simulink model "Campus_Power_System_updated"  (R2024a)
settings: Solver=daessc  StartTime=0.0  StopTime=1  RelTol=1e-3
libraries: spsThreePhaseVIMeasurementLib x57, spsThreePhaseTransformerTwoWindingsLib x56, spsThreePhaseSeriesRLCLoadLib x55, spsThreePhasePISectionLineLib x54, spsThreePhaseBreakerLib x9, spsCurrentMeasurementLib x3, spsMultimeterLib x1, spsThreePhaseSourceLib x1, spsThreePhaseFaultLib x1, sps_lib x1
(part 3 of 3)

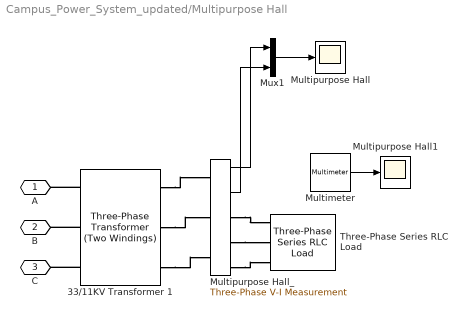
== system Campus_Power_System_updated/Multipurpose Hall ==
  33/11KV Transformer 1 : spsThreePhaseTransformerTwoWindingsLib/Three-Phase Transformer (Two Windings)  Winding1Connection=Yg  Winding2Connection=Yg  CoreType=Three single-phase transformers  SetSaturation=off  Hysteresis=off  DataFile='hysteresis'  SetInitialFlux=off  Measurements=None  UNITS=pu  NominalPower=[ 250e6 , 50 ]  Winding1=[33e3 , 0.002 , 0.08 ]  Winding2=[ 11e3 , 0.002 , 0.08 ]  Rm=500  Lm=500  L0=0.5  Saturation=[ 0,0 ; 0.0024,1.2 ; 1.0,1.52 ]  InitialFluxes=[ 0.8 , -0.8 , 0.7 ]  BreakLoop=off  DiscreteSolver=Trapezoidal iterative  DataType=off  TransfoNumber=1
  Multimeter : spsMultimeterLib/Multimeter  L=21  sel=[4 5 6]  yselected={}  Gain=[1 1 1]  OutputType=Complex  PlotAtSimulationStop=off  PhasorSimulation=off
  Multipurpose Hall : Scope
  Multipurpose Hall1 : Scope
  Multipurpose Hall_ : spsThreePhaseVIMeasurementLib/Three-Phase V-I Measurement  VoltageMeasurement=phase-to-ground  SetLabelV=off  LabelV=Vabc  Vpu=off  VpuLL=off  CurrentMeasurement=yes  SetLabelI=off  LabelI=Iabc  Ipu=off  Pbase=100e6  Vbase=500e3  OutputType=Complex  PhasorSimulation=off  PSBequivalent=0
  Mux1 : Mux  Inputs=2
  Three-Phase Series RLC Load : spsThreePhaseSeriesRLCLoadLib/Three-Phase Series RLC Load  LConnTagsString=A|B|C  Configuration=Y (grounded)  NominalVoltage=230  Vabc=[1e3 1e3 1e3]  Vabcp=[1e3 1e3 1e3]  NominalFrequency=50  UnbalancedPower=off  ActivePower=120e3  InductivePower=100  CapacitivePower=100  Pabc=[10e3 9e3 11e3]  QLabc=[100 90 110]  QCabc=[100 90 110]  Pabcp=[10e3 9e3 11e3]  QLabcp=[100 90 110]  QCabcp=[100 90 110]  Measurements=Branch currents  LoadType=constant Z
  A : PMIOPort  Side=Left
  B : PMIOPort  Port=2  Side=Left
  C : PMIOPort  Port=3  Side=Left
  wires:
  Multipurpose Hall_/2 -> Mux1/2
  Multipurpose Hall_/1 -> Mux1/1
  Mux1/1 -> Multipurpose Hall/1
  Multimeter/1 -> Multipurpose Hall1/1
  connections:
  33/11KV Transformer 1/RConn3 -- Multipurpose Hall_/LConn3
  33/11KV Transformer 1/RConn1 -- Multipurpose Hall_/LConn1
  Multipurpose Hall_/RConn2 -- Three-Phase Series RLC Load/LConn2
  Multipurpose Hall_/RConn3 -- Three-Phase Series RLC Load/LConn3
  33/11KV Transformer 1/RConn2 -- Multipurpose Hall_/LConn2
  Multipurpose Hall_/RConn1 -- Three-Phase Series RLC Load/LConn1
  33/11KV Transformer 1/LConn1 -- A/RConn1
  33/11KV Transformer 1/LConn3 -- C/RConn1
  33/11KV Transformer 1/LConn2 -- B/RConn1

== system Campus_Power_System_updated/Ogenge Odo ==
  33/11KV Transformer 1 : spsThreePhaseTransformerTwoWindingsLib/Three-Phase Transformer (Two Windings)  Winding1Connection=Yg  Winding2Connection=Yg  CoreType=Three single-phase transformers  SetSaturation=off  Hysteresis=off  DataFile='hysteresis'  SetInitialFlux=off  Measurements=None  UNITS=pu  NominalPower=[ 250e6 , 50 ]  Winding1=[33e3 , 0.002 , 0.08 ]  Winding2=[ 11e3 , 0.002 , 0.08 ]  Rm=500  Lm=500  L0=0.5  Saturation=[ 0,0 ; 0.0024,1.2 ; 1.0,1.52 ]  InitialFluxes=[ 0.8 , -0.8 , 0.7 ]  BreakLoop=off  DiscreteSolver=Trapezoidal iterative  DataType=off  TransfoNumber=1
  BUS1 : spsThreePhaseVIMeasurementLib/Three-Phase V-I Measurement  VoltageMeasurement=phase-to-ground  SetLabelV=off  LabelV=Vabc  Vpu=off  VpuLL=off  CurrentMeasurement=yes  SetLabelI=off  LabelI=Iabc  Ipu=off  Pbase=100e6  Vbase=500e3  OutputType=Complex  PhasorSimulation=off  PSBequivalent=0
  Mux1 : Mux  Inputs=2
  Scope1 : Scope
  Three-Phase Series RLC Load : spsThreePhaseSeriesRLCLoadLib/Three-Phase Series RLC Load  LConnTagsString=A|B|C  Configuration=Y (grounded)  NominalVoltage=1000  Vabc=[1e3 1e3 1e3]  Vabcp=[1e3 1e3 1e3]  NominalFrequency=60  UnbalancedPower=off  ActivePower=10e3  InductivePower=100  CapacitivePower=100  Pabc=[10e3 9e3 11e3]  QLabc=[100 90 110]  QCabc=[100 90 110]  Pabcp=[10e3 9e3 11e3]  QLabcp=[100 90 110]  QCabcp=[100 90 110]  Measurements=None  LoadType=constant Z
  A : PMIOPort  Side=Left
  B : PMIOPort  Port=2  Side=Left
  C : PMIOPort  Port=3  Side=Left
  wires:
  BUS1/2 -> Mux1/2
  BUS1/1 -> Mux1/1
  Mux1/1 -> Scope1/1
  connections:
  33/11KV Transformer 1/RConn3 -- BUS1/LConn3
  33/11KV Transformer 1/RConn1 -- BUS1/LConn1
  BUS1/RConn2 -- Three-Phase Series RLC Load/LConn2
  BUS1/RConn3 -- Three-Phase Series RLC Load/LConn3
  33/11KV Transformer 1/RConn2 -- BUS1/LConn2
  BUS1/RConn1 -- Three-Phase Series RLC Load/LConn1
  33/11KV Transformer 1/LConn1 -- A/RConn1
  33/11KV Transformer 1/LConn3 -- C/RConn1
  33/11KV Transformer 1/LConn2 -- B/RConn1

== system Campus_Power_System_updated/Ozukar Road ==
  33/11KV Transformer 1 : spsThreePhaseTransformerTwoWindingsLib/Three-Phase Transformer (Two Windings)  Winding1Connection=Yg  Winding2Connection=Yg  CoreType=Three single-phase transformers  SetSaturation=off  Hysteresis=off  DataFile='hysteresis'  SetInitialFlux=off  Measurements=None  UNITS=pu  NominalPower=[ 250e6 , 50 ]  Winding1=[33e3 , 0.002 , 0.08 ]  Winding2=[ 11e3 , 0.002 , 0.08 ]  Rm=500  Lm=500  L0=0.5  Saturation=[ 0,0 ; 0.0024,1.2 ; 1.0,1.52 ]  InitialFluxes=[ 0.8 , -0.8 , 0.7 ]  BreakLoop=off  DiscreteSolver=Trapezoidal iterative  DataType=off  TransfoNumber=1
  BUS1 : spsThreePhaseVIMeasurementLib/Three-Phase V-I Measurement  VoltageMeasurement=phase-to-ground  SetLabelV=off  LabelV=Vabc  Vpu=off  VpuLL=off  CurrentMeasurement=yes  SetLabelI=off  LabelI=Iabc  Ipu=off  Pbase=100e6  Vbase=500e3  OutputType=Complex  PhasorSimulation=off  PSBequivalent=0
  Mux1 : Mux  Inputs=2
  Scope1 : Scope
  Three-Phase Series RLC Load : spsThreePhaseSeriesRLCLoadLib/Three-Phase Series RLC Load  LConnTagsString=A|B|C  Configuration=Y (grounded)  NominalVoltage=1000  Vabc=[1e3 1e3 1e3]  Vabcp=[1e3 1e3 1e3]  NominalFrequency=60  UnbalancedPower=off  ActivePower=10e3  InductivePower=100  CapacitivePower=100  Pabc=[10e3 9e3 11e3]  QLabc=[100 90 110]  QCabc=[100 90 110]  Pabcp=[10e3 9e3 11e3]  QLabcp=[100 90 110]  QCabcp=[100 90 110]  Measurements=None  LoadType=constant Z
  A : PMIOPort  Side=Left
  B : PMIOPort  Port=2  Side=Left
  C : PMIOPort  Port=3  Side=Left
  wires:
  BUS1/2 -> Mux1/2
  BUS1/1 -> Mux1/1
  Mux1/1 -> Scope1/1
  connections:
  33/11KV Transformer 1/RConn3 -- BUS1/LConn3
  33/11KV Transformer 1/RConn1 -- BUS1/LConn1
  BUS1/RConn2 -- Three-Phase Series RLC Load/LConn2
  BUS1/RConn3 -- Three-Phase Series RLC Load/LConn3
  33/11KV Transformer 1/RConn2 -- BUS1/LConn2
  BUS1/RConn1 -- Three-Phase Series RLC Load/LConn1
  33/11KV Transformer 1/LConn1 -- A/RConn1
  33/11KV Transformer 1/LConn3 -- C/RConn1
  33/11KV Transformer 1/LConn2 -- B/RConn1

== system Campus_Power_System_updated/Place of worship ==
  33/11KV Transformer 1 : spsThreePhaseTransformerTwoWindingsLib/Three-Phase Transformer (Two Windings)  Winding1Connection=Yg  Winding2Connection=Yg  CoreType=Three single-phase transformers  SetSaturation=off  Hysteresis=off  DataFile='hysteresis'  SetInitialFlux=off  Measurements=None  UNITS=pu  NominalPower=[ 250e6 , 50 ]  Winding1=[33e3 , 0.002 , 0.08 ]  Winding2=[ 11e3 , 0.002 , 0.08 ]  Rm=500  Lm=500  L0=0.5  Saturation=[ 0,0 ; 0.0024,1.2 ; 1.0,1.52 ]  InitialFluxes=[ 0.8 , -0.8 , 0.7 ]  BreakLoop=off  DiscreteSolver=Trapezoidal iterative  DataType=off  TransfoNumber=1
  Mux1 : Mux  Inputs=2
  Place of worship : Scope
  Place of worship_ : spsThreePhaseVIMeasurementLib/Three-Phase V-I Measurement  VoltageMeasurement=phase-to-ground  SetLabelV=off  LabelV=Vabc  Vpu=off  VpuLL=off  CurrentMeasurement=yes  SetLabelI=off  LabelI=Iabc  Ipu=off  Pbase=100e6  Vbase=500e3  OutputType=Complex  PhasorSimulation=off  PSBequivalent=0
  Three-Phase Series RLC Load : spsThreePhaseSeriesRLCLoadLib/Three-Phase Series RLC Load  LConnTagsString=A|B|C  Configuration=Y (grounded)  NominalVoltage=220  Vabc=[1e3 1e3 1e3]  Vabcp=[1e3 1e3 1e3]  NominalFrequency=50  UnbalancedPower=off  ActivePower=50e3  InductivePower=100  CapacitivePower=100  Pabc=[10e3 9e3 11e3]  QLabc=[100 90 110]  QCabc=[100 90 110]  Pabcp=[10e3 9e3 11e3]  QLabcp=[100 90 110]  QCabcp=[100 90 110]  Measurements=None  LoadType=constant Z
  A : PMIOPort  Side=Left
  B : PMIOPort  Port=2  Side=Left
  C : PMIOPort  Port=3  Side=Left
  wires:
  Place of worship_/2 -> Mux1/2
  Place of worship_/1 -> Mux1/1
  Mux1/1 -> Place of worship/1
  connections:
  33/11KV Transformer 1/RConn3 -- Place of worship_/LConn3
  33/11KV Transformer 1/RConn1 -- Place of worship_/LConn1
  Place of worship_/RConn2 -- Three-Phase Series RLC Load/LConn2
  Place of worship_/RConn3 -- Three-Phase Series RLC Load/LConn3
  33/11KV Transformer 1/RConn2 -- Place of worship_/LConn2
  Place of worship_/RConn1 -- Three-Phase Series RLC Load/LConn1
  33/11KV Transformer 1/LConn1 -- A/RConn1
  33/11KV Transformer 1/LConn3 -- C/RConn1
  33/11KV Transformer 1/LConn2 -- B/RConn1

== system Campus_Power_System_updated/Professor's Quarters ==
  33/11KV Transformer 1 : spsThreePhaseTransformerTwoWindingsLib/Three-Phase Transformer (Two Windings)  Winding1Connection=Yg  Winding2Connection=Yg  CoreType=Three single-phase transformers  SetSaturation=off  Hysteresis=off  DataFile='hysteresis'  SetInitialFlux=off  Measurements=None  UNITS=pu  NominalPower=[ 250e6 , 50 ]  Winding1=[33e3 , 0.002 , 0.08 ]  Winding2=[ 11e3 , 0.002 , 0.08 ]  Rm=500  Lm=500  L0=0.5  Saturation=[ 0,0 ; 0.0024,1.2 ; 1.0,1.52 ]  InitialFluxes=[ 0.8 , -0.8 , 0.7 ]  BreakLoop=off  DiscreteSolver=Trapezoidal iterative  DataType=off  TransfoNumber=1
  BUS1 : spsThreePhaseVIMeasurementLib/Three-Phase V-I Measurement  VoltageMeasurement=phase-to-ground  SetLabelV=off  LabelV=Vabc  Vpu=off  VpuLL=off  CurrentMeasurement=yes  SetLabelI=off  LabelI=Iabc  Ipu=off  Pbase=100e6  Vbase=500e3  OutputType=Complex  PhasorSimulation=off  PSBequivalent=0
  Mux1 : Mux  Inputs=2
  Scope1 : Scope
  Three-Phase Series RLC Load : spsThreePhaseSeriesRLCLoadLib/Three-Phase Series RLC Load  LConnTagsString=A|B|C  Configuration=Y (grounded)  NominalVoltage=1000  Vabc=[1e3 1e3 1e3]  Vabcp=[1e3 1e3 1e3]  NominalFrequency=60  UnbalancedPower=off  ActivePower=10e3  InductivePower=100  CapacitivePower=100  Pabc=[10e3 9e3 11e3]  QLabc=[100 90 110]  QCabc=[100 90 110]  Pabcp=[10e3 9e3 11e3]  QLabcp=[100 90 110]  QCabcp=[100 90 110]  Measurements=None  LoadType=constant Z
  A : PMIOPort  Side=Left
  B : PMIOPort  Port=2  Side=Left
  C : PMIOPort  Port=3  Side=Left
  wires:
  BUS1/2 -> Mux1/2
  BUS1/1 -> Mux1/1
  Mux1/1 -> Scope1/1
  connections:
  33/11KV Transformer 1/RConn3 -- BUS1/LConn3
  33/11KV Transformer 1/RConn1 -- BUS1/LConn1
  BUS1/RConn2 -- Three-Phase Series RLC Load/LConn2
  BUS1/RConn3 -- Three-Phase Series RLC Load/LConn3
  33/11KV Transformer 1/RConn2 -- BUS1/LConn2
  BUS1/RConn1 -- Three-Phase Series RLC Load/LConn1
  33/11KV Transformer 1/LConn1 -- A/RConn1
  33/11KV Transformer 1/LConn3 -- C/RConn1
  33/11KV Transformer 1/LConn2 -- B/RConn1

== system Campus_Power_System_updated/Proposed RMU for Environmental ==
  33/11KV Transformer 1 : spsThreePhaseTransformerTwoWindingsLib/Three-Phase Transformer (Two Windings)  Winding1Connection=Yg  Winding2Connection=Yg  CoreType=Three single-phase transformers  SetSaturation=off  Hysteresis=off  DataFile='hysteresis'  SetInitialFlux=off  Measurements=None  UNITS=pu  NominalPower=[ 250e6 , 50 ]  Winding1=[33e3 , 0.002 , 0.08 ]  Winding2=[ 11e3 , 0.002 , 0.08 ]  Rm=500  Lm=500  L0=0.5  Saturation=[ 0,0 ; 0.0024,1.2 ; 1.0,1.52 ]  InitialFluxes=[ 0.8 , -0.8 , 0.7 ]  BreakLoop=off  DiscreteSolver=Trapezoidal iterative  DataType=off  TransfoNumber=1
  Mux1 : Mux  Inputs=2
  Proposed RMU for Environmental : Scope
  Proposed RMU for Environmental_ : spsThreePhaseVIMeasurementLib/Three-Phase V-I Measurement  VoltageMeasurement=phase-to-ground  SetLabelV=off  LabelV=Vabc  Vpu=off  VpuLL=off  CurrentMeasurement=yes  SetLabelI=off  LabelI=Iabc  Ipu=off  Pbase=100e6  Vbase=500e3  OutputType=Complex  PhasorSimulation=off  PSBequivalent=0
  Three-Phase Series RLC Load : spsThreePhaseSeriesRLCLoadLib/Three-Phase Series RLC Load  LConnTagsString=A|B|C  Configuration=Y (grounded)  NominalVoltage=220  Vabc=[1e3 1e3 1e3]  Vabcp=[1e3 1e3 1e3]  NominalFrequency=50  UnbalancedPower=off  ActivePower=60e3  InductivePower=100  CapacitivePower=100  Pabc=[10e3 9e3 11e3]  QLabc=[100 90 110]  QCabc=[100 90 110]  Pabcp=[10e3 9e3 11e3]  QLabcp=[100 90 110]  QCabcp=[100 90 110]  Measurements=None  LoadType=constant Z
  A : PMIOPort  Side=Left
  B : PMIOPort  Port=2  Side=Left
  C : PMIOPort  Port=3  Side=Left
  wires:
  Proposed RMU for Environmental_/2 -> Mux1/2
  Proposed RMU for Environmental_/1 -> Mux1/1
  Mux1/1 -> Proposed RMU for Environmental/1
  connections:
  33/11KV Transformer 1/RConn3 -- Proposed RMU for Environmental_/LConn3
  33/11KV Transformer 1/RConn1 -- Proposed RMU for Environmental_/LConn1
  Proposed RMU for Environmental_/RConn2 -- Three-Phase Series RLC Load/LConn2
  Proposed RMU for Environmental_/RConn3 -- Three-Phase Series RLC Load/LConn3
  33/11KV Transformer 1/RConn2 -- Proposed RMU for Environmental_/LConn2
  Proposed RMU for Environmental_/RConn1 -- Three-Phase Series RLC Load/LConn1
  33/11KV Transformer 1/LConn1 -- A/RConn1
  33/11KV Transformer 1/LConn3 -- C/RConn1
  33/11KV Transformer 1/LConn2 -- B/RConn1

== system Campus_Power_System_updated/RMU ==
  33/11KV Transformer 1 : spsThreePhaseTransformerTwoWindingsLib/Three-Phase Transformer (Two Windings)  Winding1Connection=Yg  Winding2Connection=Yg  CoreType=Three single-phase transformers  SetSaturation=off  Hysteresis=off  DataFile='hysteresis'  SetInitialFlux=off  Measurements=None  UNITS=pu  NominalPower=[ 250e6 , 50 ]  Winding1=[33e3 , 0.002 , 0.08 ]  Winding2=[ 11e3 , 0.002 , 0.08 ]  Rm=500  Lm=500  L0=0.5  Saturation=[ 0,0 ; 0.0024,1.2 ; 1.0,1.52 ]  InitialFluxes=[ 0.8 , -0.8 , 0.7 ]  BreakLoop=off  DiscreteSolver=Trapezoidal iterative  DataType=off  TransfoNumber=1
  BUS1 : spsThreePhaseVIMeasurementLib/Three-Phase V-I Measurement  VoltageMeasurement=phase-to-ground  SetLabelV=off  LabelV=Vabc  Vpu=off  VpuLL=off  CurrentMeasurement=yes  SetLabelI=off  LabelI=Iabc  Ipu=off  Pbase=100e6  Vbase=500e3  OutputType=Complex  PhasorSimulation=off  PSBequivalent=0
  Mux1 : Mux  Inputs=2
  Scope1 : Scope
  Three-Phase Series RLC Load : spsThreePhaseSeriesRLCLoadLib/Three-Phase Series RLC Load  LConnTagsString=A|B|C  Configuration=Y (grounded)  NominalVoltage=1000  Vabc=[1e3 1e3 1e3]  Vabcp=[1e3 1e3 1e3]  NominalFrequency=60  UnbalancedPower=off  ActivePower=10e3  InductivePower=100  CapacitivePower=100  Pabc=[10e3 9e3 11e3]  QLabc=[100 90 110]  QCabc=[100 90 110]  Pabcp=[10e3 9e3 11e3]  QLabcp=[100 90 110]  QCabcp=[100 90 110]  Measurements=None  LoadType=constant Z
  A : PMIOPort  Side=Left
  B : PMIOPort  Port=2  Side=Left
  C : PMIOPort  Port=3  Side=Left
  wires:
  BUS1/2 -> Mux1/2
  BUS1/1 -> Mux1/1
  Mux1/1 -> Scope1/1
  connections:
  33/11KV Transformer 1/RConn3 -- BUS1/LConn3
  33/11KV Transformer 1/RConn1 -- BUS1/LConn1
  BUS1/RConn2 -- Three-Phase Series RLC Load/LConn2
  BUS1/RConn3 -- Three-Phase Series RLC Load/LConn3
  33/11KV Transformer 1/RConn2 -- BUS1/LConn2
  BUS1/RConn1 -- Three-Phase Series RLC Load/LConn1
  33/11KV Transformer 1/LConn1 -- A/RConn1
  33/11KV Transformer 1/LConn3 -- C/RConn1
  33/11KV Transformer 1/LConn2 -- B/RConn1

== system Campus_Power_System_updated/Ransome Kuti Quarters ==
  33/11KV Transformer 1 : spsThreePhaseTransformerTwoWindingsLib/Three-Phase Transformer (Two Windings)  Winding1Connection=Yg  Winding2Connection=Yg  CoreType=Three single-phase transformers  SetSaturation=off  Hysteresis=off  DataFile='hysteresis'  SetInitialFlux=off  Measurements=None  UNITS=pu  NominalPower=[ 250e6 , 50 ]  Winding1=[33e3 , 0.002 , 0.08 ]  Winding2=[ 11e3 , 0.002 , 0.08 ]  Rm=500  Lm=500  L0=0.5  Saturation=[ 0,0 ; 0.0024,1.2 ; 1.0,1.52 ]  InitialFluxes=[ 0.8 , -0.8 , 0.7 ]  BreakLoop=off  DiscreteSolver=Trapezoidal iterative  DataType=off  TransfoNumber=1
  BUS1 : spsThreePhaseVIMeasurementLib/Three-Phase V-I Measurement  VoltageMeasurement=phase-to-ground  SetLabelV=off  LabelV=Vabc  Vpu=off  VpuLL=off  CurrentMeasurement=yes  SetLabelI=off  LabelI=Iabc  Ipu=off  Pbase=100e6  Vbase=500e3  OutputType=Complex  PhasorSimulation=off  PSBequivalent=0
  Mux1 : Mux  Inputs=2
  Scope1 : Scope
  Three-Phase Series RLC Load : spsThreePhaseSeriesRLCLoadLib/Three-Phase Series RLC Load  LConnTagsString=A|B|C  Configuration=Y (grounded)  NominalVoltage=1000  Vabc=[1e3 1e3 1e3]  Vabcp=[1e3 1e3 1e3]  NominalFrequency=60  UnbalancedPower=off  ActivePower=10e3  InductivePower=100  CapacitivePower=100  Pabc=[10e3 9e3 11e3]  QLabc=[100 90 110]  QCabc=[100 90 110]  Pabcp=[10e3 9e3 11e3]  QLabcp=[100 90 110]  QCabcp=[100 90 110]  Measurements=None  LoadType=constant Z
  A : PMIOPort  Side=Left
  B : PMIOPort  Port=2  Side=Left
  C : PMIOPort  Port=3  Side=Left
  wires:
  BUS1/2 -> Mux1/2
  BUS1/1 -> Mux1/1
  Mux1/1 -> Scope1/1
  connections:
  33/11KV Transformer 1/RConn3 -- BUS1/LConn3
  33/11KV Transformer 1/RConn1 -- BUS1/LConn1
  BUS1/RConn2 -- Three-Phase Series RLC Load/LConn2
  BUS1/RConn3 -- Three-Phase Series RLC Load/LConn3
  33/11KV Transformer 1/RConn2 -- BUS1/LConn2
  BUS1/RConn1 -- Three-Phase Series RLC Load/LConn1
  33/11KV Transformer 1/LConn1 -- A/RConn1
  33/11KV Transformer 1/LConn3 -- C/RConn1
  33/11KV Transformer 1/LConn2 -- B/RConn1

== system Campus_Power_System_updated/Science Complex N ==
  33/11KV Transformer 1 : spsThreePhaseTransformerTwoWindingsLib/Three-Phase Transformer (Two Windings)  Winding1Connection=Yg  Winding2Connection=Yg  CoreType=Three single-phase transformers  SetSaturation=off  Hysteresis=off  DataFile='hysteresis'  SetInitialFlux=off  Measurements=None  UNITS=pu  NominalPower=[ 250e6 , 50 ]  Winding1=[33e3 , 0.002 , 0.08 ]  Winding2=[ 11e3 , 0.002 , 0.08 ]  Rm=500  Lm=500  L0=0.5  Saturation=[ 0,0 ; 0.0024,1.2 ; 1.0,1.52 ]  InitialFluxes=[ 0.8 , -0.8 , 0.7 ]  BreakLoop=off  DiscreteSolver=Trapezoidal iterative  DataType=off  TransfoNumber=1
  BUS1 : spsThreePhaseVIMeasurementLib/Three-Phase V-I Measurement  VoltageMeasurement=phase-to-ground  SetLabelV=off  LabelV=Vabc  Vpu=off  VpuLL=off  CurrentMeasurement=yes  SetLabelI=off  LabelI=Iabc  Ipu=off  Pbase=100e6  Vbase=500e3  OutputType=Complex  PhasorSimulation=off  PSBequivalent=0
  Mux1 : Mux  Inputs=2
  Scope1 : Scope
  Three-Phase Series RLC Load : spsThreePhaseSeriesRLCLoadLib/Three-Phase Series RLC Load  LConnTagsString=A|B|C  Configuration=Y (grounded)  NominalVoltage=1000  Vabc=[1e3 1e3 1e3]  Vabcp=[1e3 1e3 1e3]  NominalFrequency=60  UnbalancedPower=off  ActivePower=10e3  InductivePower=100  CapacitivePower=100  Pabc=[10e3 9e3 11e3]  QLabc=[100 90 110]  QCabc=[100 90 110]  Pabcp=[10e3 9e3 11e3]  QLabcp=[100 90 110]  QCabcp=[100 90 110]  Measurements=None  LoadType=constant Z
  A : PMIOPort  Side=Left
  B : PMIOPort  Port=2  Side=Left
  C : PMIOPort  Port=3  Side=Left
  wires:
  BUS1/2 -> Mux1/2
  BUS1/1 -> Mux1/1
  Mux1/1 -> Scope1/1
  connections:
  33/11KV Transformer 1/RConn3 -- BUS1/LConn3
  33/11KV Transformer 1/RConn1 -- BUS1/LConn1
  BUS1/RConn2 -- Three-Phase Series RLC Load/LConn2
  BUS1/RConn3 -- Three-Phase Series RLC Load/LConn3
  33/11KV Transformer 1/RConn2 -- BUS1/LConn2
  BUS1/RConn1 -- Three-Phase Series RLC Load/LConn1
  33/11KV Transformer 1/LConn1 -- A/RConn1
  33/11KV Transformer 1/LConn3 -- C/RConn1
  33/11KV Transformer 1/LConn2 -- B/RConn1

== system Campus_Power_System_updated/Science Conplex S ==
  33/11KV Transformer 1 : spsThreePhaseTransformerTwoWindingsLib/Three-Phase Transformer (Two Windings)  Winding1Connection=Yg  Winding2Connection=Yg  CoreType=Three single-phase transformers  SetSaturation=off  Hysteresis=off  DataFile='hysteresis'  SetInitialFlux=off  Measurements=None  UNITS=pu  NominalPower=[ 250e6 , 50 ]  Winding1=[33e3 , 0.002 , 0.08 ]  Winding2=[ 11e3 , 0.002 , 0.08 ]  Rm=500  Lm=500  L0=0.5  Saturation=[ 0,0 ; 0.0024,1.2 ; 1.0,1.52 ]  InitialFluxes=[ 0.8 , -0.8 , 0.7 ]  BreakLoop=off  DiscreteSolver=Trapezoidal iterative  DataType=off  TransfoNumber=1
  BUS1 : spsThreePhaseVIMeasurementLib/Three-Phase V-I Measurement  VoltageMeasurement=phase-to-ground  SetLabelV=off  LabelV=Vabc  Vpu=off  VpuLL=off  CurrentMeasurement=yes  SetLabelI=off  LabelI=Iabc  Ipu=off  Pbase=100e6  Vbase=500e3  OutputType=Complex  PhasorSimulation=off  PSBequivalent=0
  Mux1 : Mux  Inputs=2
  Scope1 : Scope
  Three-Phase Series RLC Load : spsThreePhaseSeriesRLCLoadLib/Three-Phase Series RLC Load  LConnTagsString=A|B|C  Configuration=Y (grounded)  NominalVoltage=1000  Vabc=[1e3 1e3 1e3]  Vabcp=[1e3 1e3 1e3]  NominalFrequency=60  UnbalancedPower=off  ActivePower=10e3  InductivePower=100  CapacitivePower=100  Pabc=[10e3 9e3 11e3]  QLabc=[100 90 110]  QCabc=[100 90 110]  Pabcp=[10e3 9e3 11e3]  QLabcp=[100 90 110]  QCabcp=[100 90 110]  Measurements=None  LoadType=constant Z
  A : PMIOPort  Side=Left
  B : PMIOPort  Port=2  Side=Left
  C : PMIOPort  Port=3  Side=Left
  wires:
  BUS1/2 -> Mux1/2
  BUS1/1 -> Mux1/1
  Mux1/1 -> Scope1/1
  connections:
  33/11KV Transformer 1/RConn3 -- BUS1/LConn3
  33/11KV Transformer 1/RConn1 -- BUS1/LConn1
  BUS1/RConn2 -- Three-Phase Series RLC Load/LConn2
  BUS1/RConn3 -- Three-Phase Series RLC Load/LConn3
  33/11KV Transformer 1/RConn2 -- BUS1/LConn2
  BUS1/RConn1 -- Three-Phase Series RLC Load/LConn1
  33/11KV Transformer 1/LConn1 -- A/RConn1
  33/11KV Transformer 1/LConn3 -- C/RConn1
  33/11KV Transformer 1/LConn2 -- B/RConn1

== system Campus_Power_System_updated/Science complex E ==
  33/11KV Transformer 1 : spsThreePhaseTransformerTwoWindingsLib/Three-Phase Transformer (Two Windings)  Winding1Connection=Yg  Winding2Connection=Yg  CoreType=Three single-phase transformers  SetSaturation=off  Hysteresis=off  DataFile='hysteresis'  SetInitialFlux=off  Measurements=None  UNITS=pu  NominalPower=[ 250e6 , 50 ]  Winding1=[33e3 , 0.002 , 0.08 ]  Winding2=[ 11e3 , 0.002 , 0.08 ]  Rm=500  Lm=500  L0=0.5  Saturation=[ 0,0 ; 0.0024,1.2 ; 1.0,1.52 ]  InitialFluxes=[ 0.8 , -0.8 , 0.7 ]  BreakLoop=off  DiscreteSolver=Trapezoidal iterative  DataType=off  TransfoNumber=1
  BUS1 : spsThreePhaseVIMeasurementLib/Three-Phase V-I Measurement  VoltageMeasurement=phase-to-ground  SetLabelV=off  LabelV=Vabc  Vpu=off  VpuLL=off  CurrentMeasurement=yes  SetLabelI=off  LabelI=Iabc  Ipu=off  Pbase=100e6  Vbase=500e3  OutputType=Complex  PhasorSimulation=off  PSBequivalent=0
  Mux1 : Mux  Inputs=2
  Scope1 : Scope
  Three-Phase Series RLC Load : spsThreePhaseSeriesRLCLoadLib/Three-Phase Series RLC Load  LConnTagsString=A|B|C  Configuration=Y (grounded)  NominalVoltage=1000  Vabc=[1e3 1e3 1e3]  Vabcp=[1e3 1e3 1e3]  NominalFrequency=60  UnbalancedPower=off  ActivePower=10e3  InductivePower=100  CapacitivePower=100  Pabc=[10e3 9e3 11e3]  QLabc=[100 90 110]  QCabc=[100 90 110]  Pabcp=[10e3 9e3 11e3]  QLabcp=[100 90 110]  QCabcp=[100 90 110]  Measurements=None  LoadType=constant Z
  A : PMIOPort  Side=Left
  B : PMIOPort  Port=2  Side=Left
  C : PMIOPort  Port=3  Side=Left
  wires:
  BUS1/2 -> Mux1/2
  BUS1/1 -> Mux1/1
  Mux1/1 -> Scope1/1
  connections:
  33/11KV Transformer 1/RConn3 -- BUS1/LConn3
  33/11KV Transformer 1/RConn1 -- BUS1/LConn1
  BUS1/RConn2 -- Three-Phase Series RLC Load/LConn2
  BUS1/RConn3 -- Three-Phase Series RLC Load/LConn3
  33/11KV Transformer 1/RConn2 -- BUS1/LConn2
  BUS1/RConn1 -- Three-Phase Series RLC Load/LConn1
  33/11KV Transformer 1/LConn1 -- A/RConn1
  33/11KV Transformer 1/LConn3 -- C/RConn1
  33/11KV Transformer 1/LConn2 -- B/RConn1

== system Campus_Power_System_updated/Senate House (1) ==
  33/11KV Transformer 1 : spsThreePhaseTransformerTwoWindingsLib/Three-Phase Transformer (Two Windings)  Winding1Connection=Yg  Winding2Connection=Yg  CoreType=Three single-phase transformers  SetSaturation=off  Hysteresis=off  DataFile='hysteresis'  SetInitialFlux=off  Measurements=None  UNITS=pu  NominalPower=[ 250e6 , 50 ]  Winding1=[33e3 , 0.002 , 0.08 ]  Winding2=[ 11e3 , 0.002 , 0.08 ]  Rm=500  Lm=500  L0=0.5  Saturation=[ 0,0 ; 0.0024,1.2 ; 1.0,1.52 ]  InitialFluxes=[ 0.8 , -0.8 , 0.7 ]  BreakLoop=off  DiscreteSolver=Trapezoidal iterative  DataType=off  TransfoNumber=1
  BUS1 : spsThreePhaseVIMeasurementLib/Three-Phase V-I Measurement  VoltageMeasurement=phase-to-ground  SetLabelV=off  LabelV=Vabc  Vpu=off  VpuLL=off  CurrentMeasurement=yes  SetLabelI=off  LabelI=Iabc  Ipu=off  Pbase=100e6  Vbase=500e3  OutputType=Complex  PhasorSimulation=off  PSBequivalent=0
  Mux1 : Mux  Inputs=2
  Scope1 : Scope
  Three-Phase Series RLC Load : spsThreePhaseSeriesRLCLoadLib/Three-Phase Series RLC Load  LConnTagsString=A|B|C  Configuration=Y (grounded)  NominalVoltage=1000  Vabc=[1e3 1e3 1e3]  Vabcp=[1e3 1e3 1e3]  NominalFrequency=60  UnbalancedPower=off  ActivePower=10e3  InductivePower=100  CapacitivePower=100  Pabc=[10e3 9e3 11e3]  QLabc=[100 90 110]  QCabc=[100 90 110]  Pabcp=[10e3 9e3 11e3]  QLabcp=[100 90 110]  QCabcp=[100 90 110]  Measurements=None  LoadType=constant Z
  A : PMIOPort  Side=Left
  B : PMIOPort  Port=2  Side=Left
  C : PMIOPort  Port=3  Side=Left
  wires:
  BUS1/2 -> Mux1/2
  BUS1/1 -> Mux1/1
  Mux1/1 -> Scope1/1
  connections:
  33/11KV Transformer 1/RConn3 -- BUS1/LConn3
  33/11KV Transformer 1/RConn1 -- BUS1/LConn1
  BUS1/RConn2 -- Three-Phase Series RLC Load/LConn2
  BUS1/RConn3 -- Three-Phase Series RLC Load/LConn3
  33/11KV Transformer 1/RConn2 -- BUS1/LConn2
  BUS1/RConn1 -- Three-Phase Series RLC Load/LConn1
  33/11KV Transformer 1/LConn1 -- A/RConn1
  33/11KV Transformer 1/LConn3 -- C/RConn1
  33/11KV Transformer 1/LConn2 -- B/RConn1

== system Campus_Power_System_updated/Senate House (2) ==
  33/11KV Transformer 1 : spsThreePhaseTransformerTwoWindingsLib/Three-Phase Transformer (Two Windings)  Winding1Connection=Yg  Winding2Connection=Yg  CoreType=Three single-phase transformers  SetSaturation=off  Hysteresis=off  DataFile='hysteresis'  SetInitialFlux=off  Measurements=None  UNITS=pu  NominalPower=[ 250e6 , 50 ]  Winding1=[33e3 , 0.002 , 0.08 ]  Winding2=[ 11e3 , 0.002 , 0.08 ]  Rm=500  Lm=500  L0=0.5  Saturation=[ 0,0 ; 0.0024,1.2 ; 1.0,1.52 ]  InitialFluxes=[ 0.8 , -0.8 , 0.7 ]  BreakLoop=off  DiscreteSolver=Trapezoidal iterative  DataType=off  TransfoNumber=1
  BUS1 : spsThreePhaseVIMeasurementLib/Three-Phase V-I Measurement  VoltageMeasurement=phase-to-ground  SetLabelV=off  LabelV=Vabc  Vpu=off  VpuLL=off  CurrentMeasurement=yes  SetLabelI=off  LabelI=Iabc  Ipu=off  Pbase=100e6  Vbase=500e3  OutputType=Complex  PhasorSimulation=off  PSBequivalent=0
  Mux1 : Mux  Inputs=2
  Scope1 : Scope
  Three-Phase Series RLC Load : spsThreePhaseSeriesRLCLoadLib/Three-Phase Series RLC Load  LConnTagsString=A|B|C  Configuration=Y (grounded)  NominalVoltage=1000  Vabc=[1e3 1e3 1e3]  Vabcp=[1e3 1e3 1e3]  NominalFrequency=60  UnbalancedPower=off  ActivePower=10e3  InductivePower=100  CapacitivePower=100  Pabc=[10e3 9e3 11e3]  QLabc=[100 90 110]  QCabc=[100 90 110]  Pabcp=[10e3 9e3 11e3]  QLabcp=[100 90 110]  QCabcp=[100 90 110]  Measurements=None  LoadType=constant Z
  A : PMIOPort  Side=Left
  B : PMIOPort  Port=2  Side=Left
  C : PMIOPort  Port=3  Side=Left
  wires:
  BUS1/2 -> Mux1/2
  BUS1/1 -> Mux1/1
  Mux1/1 -> Scope1/1
  connections:
  33/11KV Transformer 1/RConn3 -- BUS1/LConn3
  33/11KV Transformer 1/RConn1 -- BUS1/LConn1
  BUS1/RConn2 -- Three-Phase Series RLC Load/LConn2
  BUS1/RConn3 -- Three-Phase Series RLC Load/LConn3
  33/11KV Transformer 1/RConn2 -- BUS1/LConn2
  BUS1/RConn1 -- Three-Phase Series RLC Load/LConn1
  33/11KV Transformer 1/LConn1 -- A/RConn1
  33/11KV Transformer 1/LConn3 -- C/RConn1
  33/11KV Transformer 1/LConn2 -- B/RConn1

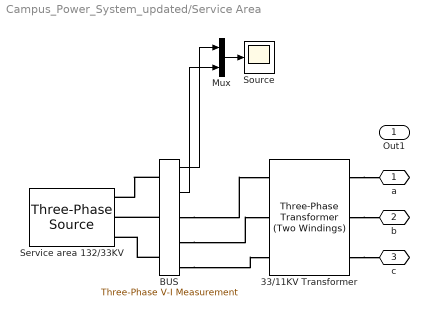
== system Campus_Power_System_updated/Service Area ==
  "33/11KV Transformer " : spsThreePhaseTransformerTwoWindingsLib/Three-Phase Transformer (Two Windings)  Winding1Connection=Yg  Winding2Connection=Yg  CoreType=Three single-phase transformers  SetSaturation=off  Hysteresis=off  DataFile='hysteresis'  SetInitialFlux=off  Measurements=None  UNITS=pu  NominalPower=[ 250e6 , 50 ]  Winding1=[33e3 , 0.002 , 0.08 ]  Winding2=[ 11e3 , 0.002 , 0.08 ]  Rm=500  Lm=500  L0=0.5  Saturation=[ 0,0 ; 0.0024,1.2 ; 1.0,1.52 ]  InitialFluxes=[ 0.8 , -0.8 , 0.7 ]  BreakLoop=off  DiscreteSolver=Trapezoidal iterative  DataType=off  TransfoNumber=1
  BUS : spsThreePhaseVIMeasurementLib/Three-Phase V-I Measurement  VoltageMeasurement=phase-to-ground  SetLabelV=off  LabelV=Vabc  Vpu=off  VpuLL=off  CurrentMeasurement=yes  SetLabelI=off  LabelI=Iabc  Ipu=off  Pbase=100e6  Vbase=500e3  OutputType=Complex  PhasorSimulation=off  PSBequivalent=0
  Mux : Mux  Inputs=2
  Service area 132/33KV : spsThreePhaseSourceLib/Three-Phase Source  InternalConnection=Yg  VoltagePhases=off  Voltage=25e3  PhaseAngle=0  Voltage_phases=[25e3 25e3 25e3]/sqrt(3)  PhaseAngles_phases=[0 -120 +120]  Frequency=50  NonIdealSource=on  SpecifyImpedance=off  Resistance=0.1  Inductance=0.01  ShortCircuitLevel=100e6  BaseVoltage=25e3  XRratio=7  BusType=swing  Pref=10e3  Qref=0  Prefabc=[10e3, 10e3, 10e3]  Qrefabc=[0, 0, 0]  Qmin=-inf  Qmax=inf
  Source : Scope
  a : PMIOPort  Side=Right
  b : PMIOPort  Port=2  Side=Right
  c : PMIOPort  Port=3  Side=Right
  Out1 : Outport
  wires:
  Mux/1 -> Source/1
  BUS/2 -> Mux/2
  BUS/1 -> Mux/1
  connections:
  BUS/RConn1 -- "33/11KV Transformer "/LConn1
  BUS/LConn2 -- Service area 132/33KV/RConn2
  "33/11KV Transformer "/RConn2 -- b/RConn1
  BUS/LConn3 -- Service area 132/33KV/RConn3
  BUS/RConn3 -- "33/11KV Transformer "/LConn3
  BUS/LConn1 -- Service area 132/33KV/RConn1
  BUS/RConn2 -- "33/11KV Transformer "/LConn2
  "33/11KV Transformer "/RConn3 -- c/RConn1
  "33/11KV Transformer "/RConn1 -- a/RConn1

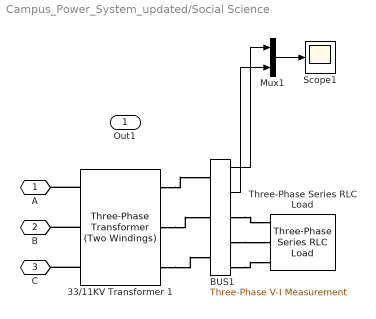
== system Campus_Power_System_updated/Social Science ==
  33/11KV Transformer 1 : spsThreePhaseTransformerTwoWindingsLib/Three-Phase Transformer (Two Windings)  Winding1Connection=Yg  Winding2Connection=Yg  CoreType=Three single-phase transformers  SetSaturation=off  Hysteresis=off  DataFile='hysteresis'  SetInitialFlux=off  Measurements=None  UNITS=pu  NominalPower=[ 250e6 , 50 ]  Winding1=[33e3 , 0.002 , 0.08 ]  Winding2=[ 11e3 , 0.002 , 0.08 ]  Rm=500  Lm=500  L0=0.5  Saturation=[ 0,0 ; 0.0024,1.2 ; 1.0,1.52 ]  InitialFluxes=[ 0.8 , -0.8 , 0.7 ]  BreakLoop=off  DiscreteSolver=Trapezoidal iterative  DataType=off  TransfoNumber=1
  BUS1 : spsThreePhaseVIMeasurementLib/Three-Phase V-I Measurement  VoltageMeasurement=phase-to-ground  SetLabelV=off  LabelV=Vabc  Vpu=off  VpuLL=off  CurrentMeasurement=yes  SetLabelI=off  LabelI=Iabc  Ipu=off  Pbase=100e6  Vbase=500e3  OutputType=Complex  PhasorSimulation=off  PSBequivalent=0
  Mux1 : Mux  Inputs=2
  Scope1 : Scope
  Three-Phase Series RLC Load : spsThreePhaseSeriesRLCLoadLib/Three-Phase Series RLC Load  LConnTagsString=A|B|C  Configuration=Y (grounded)  NominalVoltage=1000  Vabc=[1e3 1e3 1e3]  Vabcp=[1e3 1e3 1e3]  NominalFrequency=60  UnbalancedPower=off  ActivePower=10e3  InductivePower=100  CapacitivePower=100  Pabc=[10e3 9e3 11e3]  QLabc=[100 90 110]  QCabc=[100 90 110]  Pabcp=[10e3 9e3 11e3]  QLabcp=[100 90 110]  QCabcp=[100 90 110]  Measurements=None  LoadType=constant Z
  A : PMIOPort  Side=Left
  B : PMIOPort  Port=2  Side=Left
  C : PMIOPort  Port=3  Side=Left
  Out1 : Outport
  wires:
  BUS1/2 -> Mux1/2
  BUS1/1 -> Mux1/1
  Mux1/1 -> Scope1/1
  connections:
  33/11KV Transformer 1/RConn3 -- BUS1/LConn3
  33/11KV Transformer 1/RConn1 -- BUS1/LConn1
  BUS1/RConn2 -- Three-Phase Series RLC Load/LConn2
  BUS1/RConn3 -- Three-Phase Series RLC Load/LConn3
  33/11KV Transformer 1/RConn2 -- BUS1/LConn2
  BUS1/RConn1 -- Three-Phase Series RLC Load/LConn1
  33/11KV Transformer 1/LConn1 -- A/RConn1
  33/11KV Transformer 1/LConn3 -- C/RConn1
  33/11KV Transformer 1/LConn2 -- B/RConn1

== system Campus_Power_System_updated/Sport centre ==
  33/11KV Transformer 1 : spsThreePhaseTransformerTwoWindingsLib/Three-Phase Transformer (Two Windings)  Winding1Connection=Yg  Winding2Connection=Yg  CoreType=Three single-phase transformers  SetSaturation=off  Hysteresis=off  DataFile='hysteresis'  SetInitialFlux=off  Measurements=None  UNITS=pu  NominalPower=[ 250e6 , 50 ]  Winding1=[33e3 , 0.002 , 0.08 ]  Winding2=[ 11e3 , 0.002 , 0.08 ]  Rm=500  Lm=500  L0=0.5  Saturation=[ 0,0 ; 0.0024,1.2 ; 1.0,1.52 ]  InitialFluxes=[ 0.8 , -0.8 , 0.7 ]  BreakLoop=off  DiscreteSolver=Trapezoidal iterative  DataType=off  TransfoNumber=1
  BUS1 : spsThreePhaseVIMeasurementLib/Three-Phase V-I Measurement  VoltageMeasurement=phase-to-ground  SetLabelV=off  LabelV=Vabc  Vpu=off  VpuLL=off  CurrentMeasurement=yes  SetLabelI=off  LabelI=Iabc  Ipu=off  Pbase=100e6  Vbase=500e3  OutputType=Complex  PhasorSimulation=off  PSBequivalent=0
  Mux1 : Mux  Inputs=2
  Scope1 : Scope
  Three-Phase Series RLC Load : spsThreePhaseSeriesRLCLoadLib/Three-Phase Series RLC Load  LConnTagsString=A|B|C  Configuration=Y (grounded)  NominalVoltage=1000  Vabc=[1e3 1e3 1e3]  Vabcp=[1e3 1e3 1e3]  NominalFrequency=60  UnbalancedPower=off  ActivePower=10e3  InductivePower=100  CapacitivePower=100  Pabc=[10e3 9e3 11e3]  QLabc=[100 90 110]  QCabc=[100 90 110]  Pabcp=[10e3 9e3 11e3]  QLabcp=[100 90 110]  QCabcp=[100 90 110]  Measurements=None  LoadType=constant Z
  A : PMIOPort  Side=Left
  B : PMIOPort  Port=2  Side=Left
  C : PMIOPort  Port=3  Side=Left
  wires:
  BUS1/2 -> Mux1/2
  BUS1/1 -> Mux1/1
  Mux1/1 -> Scope1/1
  connections:
  33/11KV Transformer 1/RConn3 -- BUS1/LConn3
  33/11KV Transformer 1/RConn1 -- BUS1/LConn1
  BUS1/RConn2 -- Three-Phase Series RLC Load/LConn2
  BUS1/RConn3 -- Three-Phase Series RLC Load/LConn3
  33/11KV Transformer 1/RConn2 -- BUS1/LConn2
  BUS1/RConn1 -- Three-Phase Series RLC Load/LConn1
  33/11KV Transformer 1/LConn1 -- A/RConn1
  33/11KV Transformer 1/LConn3 -- C/RConn1
  33/11KV Transformer 1/LConn2 -- B/RConn1

== system Campus_Power_System_updated/Subsystem53 ==
  33/11KV Transformer 1 : spsThreePhaseTransformerTwoWindingsLib/Three-Phase Transformer (Two Windings)  Winding1Connection=Yg  Winding2Connection=Yg  CoreType=Three single-phase transformers  SetSaturation=off  Hysteresis=off  DataFile='hysteresis'  SetInitialFlux=off  Measurements=None  UNITS=pu  NominalPower=[ 250e6 , 50 ]  Winding1=[33e3 , 0.002 , 0.08 ]  Winding2=[ 11e3 , 0.002 , 0.08 ]  Rm=500  Lm=500  L0=0.5  Saturation=[ 0,0 ; 0.0024,1.2 ; 1.0,1.52 ]  InitialFluxes=[ 0.8 , -0.8 , 0.7 ]  BreakLoop=off  DiscreteSolver=Trapezoidal iterative  DataType=off  TransfoNumber=1
  BUS1 : spsThreePhaseVIMeasurementLib/Three-Phase V-I Measurement  VoltageMeasurement=phase-to-ground  SetLabelV=off  LabelV=Vabc  Vpu=off  VpuLL=off  CurrentMeasurement=yes  SetLabelI=off  LabelI=Iabc  Ipu=off  Pbase=100e6  Vbase=500e3  OutputType=Complex  PhasorSimulation=off  PSBequivalent=0
  Mux1 : Mux  Inputs=2
  Scope1 : Scope
  Three-Phase Series RLC Load : spsThreePhaseSeriesRLCLoadLib/Three-Phase Series RLC Load  LConnTagsString=A|B|C  Configuration=Y (grounded)  NominalVoltage=1000  Vabc=[1e3 1e3 1e3]  Vabcp=[1e3 1e3 1e3]  NominalFrequency=60  UnbalancedPower=off  ActivePower=10e3  InductivePower=100  CapacitivePower=100  Pabc=[10e3 9e3 11e3]  QLabc=[100 90 110]  QCabc=[100 90 110]  Pabcp=[10e3 9e3 11e3]  QLabcp=[100 90 110]  QCabcp=[100 90 110]  Measurements=None  LoadType=constant Z
  A : PMIOPort  Side=Left
  B : PMIOPort  Port=2  Side=Left
  C : PMIOPort  Port=3  Side=Left
  wires:
  BUS1/2 -> Mux1/2
  BUS1/1 -> Mux1/1
  Mux1/1 -> Scope1/1
  connections:
  33/11KV Transformer 1/RConn3 -- BUS1/LConn3
  33/11KV Transformer 1/RConn1 -- BUS1/LConn1
  BUS1/RConn2 -- Three-Phase Series RLC Load/LConn2
  BUS1/RConn3 -- Three-Phase Series RLC Load/LConn3
  33/11KV Transformer 1/RConn2 -- BUS1/LConn2
  BUS1/RConn1 -- Three-Phase Series RLC Load/LConn1
  33/11KV Transformer 1/LConn1 -- A/RConn1
  33/11KV Transformer 1/LConn3 -- C/RConn1
  33/11KV Transformer 1/LConn2 -- B/RConn1

== system Campus_Power_System_updated/Tinubu Close ==
  33/11KV Transformer 1 : spsThreePhaseTransformerTwoWindingsLib/Three-Phase Transformer (Two Windings)  Winding1Connection=Yg  Winding2Connection=Yg  CoreType=Three single-phase transformers  SetSaturation=off  Hysteresis=off  DataFile='hysteresis'  SetInitialFlux=off  Measurements=None  UNITS=pu  NominalPower=[ 250e6 , 50 ]  Winding1=[33e3 , 0.002 , 0.08 ]  Winding2=[ 11e3 , 0.002 , 0.08 ]  Rm=500  Lm=500  L0=0.5  Saturation=[ 0,0 ; 0.0024,1.2 ; 1.0,1.52 ]  InitialFluxes=[ 0.8 , -0.8 , 0.7 ]  BreakLoop=off  DiscreteSolver=Trapezoidal iterative  DataType=off  TransfoNumber=1
  BUS1 : spsThreePhaseVIMeasurementLib/Three-Phase V-I Measurement  VoltageMeasurement=phase-to-ground  SetLabelV=off  LabelV=Vabc  Vpu=off  VpuLL=off  CurrentMeasurement=yes  SetLabelI=off  LabelI=Iabc  Ipu=off  Pbase=100e6  Vbase=500e3  OutputType=Complex  PhasorSimulation=off  PSBequivalent=0
  Mux1 : Mux  Inputs=2
  Scope1 : Scope
  Three-Phase Series RLC Load : spsThreePhaseSeriesRLCLoadLib/Three-Phase Series RLC Load  LConnTagsString=A|B|C  Configuration=Y (grounded)  NominalVoltage=1000  Vabc=[1e3 1e3 1e3]  Vabcp=[1e3 1e3 1e3]  NominalFrequency=60  UnbalancedPower=off  ActivePower=10e3  InductivePower=100  CapacitivePower=100  Pabc=[10e3 9e3 11e3]  QLabc=[100 90 110]  QCabc=[100 90 110]  Pabcp=[10e3 9e3 11e3]  QLabcp=[100 90 110]  QCabcp=[100 90 110]  Measurements=None  LoadType=constant Z
  A : PMIOPort  Side=Left
  B : PMIOPort  Port=2  Side=Left
  C : PMIOPort  Port=3  Side=Left
  wires:
  BUS1/2 -> Mux1/2
  BUS1/1 -> Mux1/1
  Mux1/1 -> Scope1/1
  connections:
  33/11KV Transformer 1/RConn3 -- BUS1/LConn3
  33/11KV Transformer 1/RConn1 -- BUS1/LConn1
  BUS1/RConn2 -- Three-Phase Series RLC Load/LConn2
  BUS1/RConn3 -- Three-Phase Series RLC Load/LConn3
  33/11KV Transformer 1/RConn2 -- BUS1/LConn2
  BUS1/RConn1 -- Three-Phase Series RLC Load/LConn1
  33/11KV Transformer 1/LConn1 -- A/RConn1
  33/11KV Transformer 1/LConn3 -- C/RConn1
  33/11KV Transformer 1/LConn2 -- B/RConn1

== system Campus_Power_System_updated/Unilag Consults ==
  33/11KV Transformer 1 : spsThreePhaseTransformerTwoWindingsLib/Three-Phase Transformer (Two Windings)  Winding1Connection=Yg  Winding2Connection=Yg  CoreType=Three single-phase transformers  SetSaturation=off  Hysteresis=off  DataFile='hysteresis'  SetInitialFlux=off  Measurements=None  UNITS=pu  NominalPower=[ 250e6 , 50 ]  Winding1=[33e3 , 0.002 , 0.08 ]  Winding2=[ 11e3 , 0.002 , 0.08 ]  Rm=500  Lm=500  L0=0.5  Saturation=[ 0,0 ; 0.0024,1.2 ; 1.0,1.52 ]  InitialFluxes=[ 0.8 , -0.8 , 0.7 ]  BreakLoop=off  DiscreteSolver=Trapezoidal iterative  DataType=off  TransfoNumber=1
  BUS1 : spsThreePhaseVIMeasurementLib/Three-Phase V-I Measurement  VoltageMeasurement=phase-to-ground  SetLabelV=off  LabelV=Vabc  Vpu=off  VpuLL=off  CurrentMeasurement=yes  SetLabelI=off  LabelI=Iabc  Ipu=off  Pbase=100e6  Vbase=500e3  OutputType=Complex  PhasorSimulation=off  PSBequivalent=0
  Mux1 : Mux  Inputs=2
  Scope1 : Scope
  Three-Phase Series RLC Load : spsThreePhaseSeriesRLCLoadLib/Three-Phase Series RLC Load  LConnTagsString=A|B|C  Configuration=Y (grounded)  NominalVoltage=1000  Vabc=[1e3 1e3 1e3]  Vabcp=[1e3 1e3 1e3]  NominalFrequency=60  UnbalancedPower=off  ActivePower=10e3  InductivePower=100  CapacitivePower=100  Pabc=[10e3 9e3 11e3]  QLabc=[100 90 110]  QCabc=[100 90 110]  Pabcp=[10e3 9e3 11e3]  QLabcp=[100 90 110]  QCabcp=[100 90 110]  Measurements=None  LoadType=constant Z
  A : PMIOPort  Side=Left
  B : PMIOPort  Port=2  Side=Left
  C : PMIOPort  Port=3  Side=Left
  wires:
  BUS1/2 -> Mux1/2
  BUS1/1 -> Mux1/1
  Mux1/1 -> Scope1/1
  connections:
  33/11KV Transformer 1/RConn3 -- BUS1/LConn3
  33/11KV Transformer 1/RConn1 -- BUS1/LConn1
  BUS1/RConn2 -- Three-Phase Series RLC Load/LConn2
  BUS1/RConn3 -- Three-Phase Series RLC Load/LConn3
  33/11KV Transformer 1/RConn2 -- BUS1/LConn2
  BUS1/RConn1 -- Three-Phase Series RLC Load/LConn1
  33/11KV Transformer 1/LConn1 -- A/RConn1
  33/11KV Transformer 1/LConn3 -- C/RConn1
  33/11KV Transformer 1/LConn2 -- B/RConn1

== system Campus_Power_System_updated/VC'S Lodge ==
  33/11KV Transformer 1 : spsThreePhaseTransformerTwoWindingsLib/Three-Phase Transformer (Two Windings)  Winding1Connection=Yg  Winding2Connection=Yg  CoreType=Three single-phase transformers  SetSaturation=off  Hysteresis=off  DataFile='hysteresis'  SetInitialFlux=off  Measurements=None  UNITS=pu  NominalPower=[ 250e6 , 50 ]  Winding1=[33e3 , 0.002 , 0.08 ]  Winding2=[ 11e3 , 0.002 , 0.08 ]  Rm=500  Lm=500  L0=0.5  Saturation=[ 0,0 ; 0.0024,1.2 ; 1.0,1.52 ]  InitialFluxes=[ 0.8 , -0.8 , 0.7 ]  BreakLoop=off  DiscreteSolver=Trapezoidal iterative  DataType=off  TransfoNumber=1
  BUS1 : spsThreePhaseVIMeasurementLib/Three-Phase V-I Measurement  VoltageMeasurement=phase-to-ground  SetLabelV=off  LabelV=Vabc  Vpu=off  VpuLL=off  CurrentMeasurement=yes  SetLabelI=off  LabelI=Iabc  Ipu=off  Pbase=100e6  Vbase=500e3  OutputType=Complex  PhasorSimulation=off  PSBequivalent=0
  Mux1 : Mux  Inputs=2
  Scope1 : Scope
  Three-Phase Series RLC Load : spsThreePhaseSeriesRLCLoadLib/Three-Phase Series RLC Load  LConnTagsString=A|B|C  Configuration=Y (grounded)  NominalVoltage=1000  Vabc=[1e3 1e3 1e3]  Vabcp=[1e3 1e3 1e3]  NominalFrequency=60  UnbalancedPower=off  ActivePower=10e3  InductivePower=100  CapacitivePower=100  Pabc=[10e3 9e3 11e3]  QLabc=[100 90 110]  QCabc=[100 90 110]  Pabcp=[10e3 9e3 11e3]  QLabcp=[100 90 110]  QCabcp=[100 90 110]  Measurements=None  LoadType=constant Z
  A : PMIOPort  Side=Left
  B : PMIOPort  Port=2  Side=Left
  C : PMIOPort  Port=3  Side=Left
  wires:
  BUS1/2 -> Mux1/2
  BUS1/1 -> Mux1/1
  Mux1/1 -> Scope1/1
  connections:
  33/11KV Transformer 1/RConn3 -- BUS1/LConn3
  33/11KV Transformer 1/RConn1 -- BUS1/LConn1
  BUS1/RConn2 -- Three-Phase Series RLC Load/LConn2
  BUS1/RConn3 -- Three-Phase Series RLC Load/LConn3
  33/11KV Transformer 1/RConn2 -- BUS1/LConn2
  BUS1/RConn1 -- Three-Phase Series RLC Load/LConn1
  33/11KV Transformer 1/LConn1 -- A/RConn1
  33/11KV Transformer 1/LConn3 -- C/RConn1
  33/11KV Transformer 1/LConn2 -- B/RConn1

== system Campus_Power_System_updated/Work & Physical Planning ==
  33/11KV Transformer 1 : spsThreePhaseTransformerTwoWindingsLib/Three-Phase Transformer (Two Windings)  Winding1Connection=Yg  Winding2Connection=Yg  CoreType=Three single-phase transformers  SetSaturation=off  Hysteresis=off  DataFile='hysteresis'  SetInitialFlux=off  Measurements=None  UNITS=pu  NominalPower=[ 250e6 , 50 ]  Winding1=[33e3 , 0.002 , 0.08 ]  Winding2=[ 11e3 , 0.002 , 0.08 ]  Rm=500  Lm=500  L0=0.5  Saturation=[ 0,0 ; 0.0024,1.2 ; 1.0,1.52 ]  InitialFluxes=[ 0.8 , -0.8 , 0.7 ]  BreakLoop=off  DiscreteSolver=Trapezoidal iterative  DataType=off  TransfoNumber=1
  BUS1 : spsThreePhaseVIMeasurementLib/Three-Phase V-I Measurement  VoltageMeasurement=phase-to-ground  SetLabelV=off  LabelV=Vabc  Vpu=off  VpuLL=off  CurrentMeasurement=yes  SetLabelI=off  LabelI=Iabc  Ipu=off  Pbase=100e6  Vbase=500e3  OutputType=Complex  PhasorSimulation=off  PSBequivalent=0
  Mux1 : Mux  Inputs=2
  Scope1 : Scope
  Three-Phase Series RLC Load : spsThreePhaseSeriesRLCLoadLib/Three-Phase Series RLC Load  LConnTagsString=A|B|C  Configuration=Y (grounded)  NominalVoltage=1000  Vabc=[1e3 1e3 1e3]  Vabcp=[1e3 1e3 1e3]  NominalFrequency=60  UnbalancedPower=off  ActivePower=10e3  InductivePower=100  CapacitivePower=100  Pabc=[10e3 9e3 11e3]  QLabc=[100 90 110]  QCabc=[100 90 110]  Pabcp=[10e3 9e3 11e3]  QLabcp=[100 90 110]  QCabcp=[100 90 110]  Measurements=None  LoadType=constant Z
  A : PMIOPort  Side=Left
  B : PMIOPort  Port=2  Side=Left
  C : PMIOPort  Port=3  Side=Left
  wires:
  BUS1/2 -> Mux1/2
  BUS1/1 -> Mux1/1
  Mux1/1 -> Scope1/1
  connections:
  33/11KV Transformer 1/RConn3 -- BUS1/LConn3
  33/11KV Transformer 1/RConn1 -- BUS1/LConn1
  BUS1/RConn2 -- Three-Phase Series RLC Load/LConn2
  BUS1/RConn3 -- Three-Phase Series RLC Load/LConn3
  33/11KV Transformer 1/RConn2 -- BUS1/LConn2
  BUS1/RConn1 -- Three-Phase Series RLC Load/LConn1
  33/11KV Transformer 1/LConn1 -- A/RConn1
  33/11KV Transformer 1/LConn3 -- C/RConn1
  33/11KV Transformer 1/LConn2 -- B/RConn1

== matlab function Campus_Power_System_updated/MATLAB Function ==
  data: Ia input; breaker_cmd output; Ib input; Ic input
function breaker_cmd = simple_plc(Ia, Ib, Ic)
% Simple overcurrent protection
persistent breaker_state
if isempty(breaker_state)
    breaker_state = 1;
end

I_max = max([abs(Ia), abs(Ib), abs(Ic)]);
if I_max > 1000  % Threshold
    breaker_state = 0;  % Open breaker
end

breaker_cmd = breaker_state;
end
